simulink model "Project2"  (Simulink 8.0)
settings: Solver=ode23s  StartTime=0.0  StopTime=600  RelTol=1e-4
values from neighbouring files (symbols this model uses):
  a_1 = X(1)    [Init_Project1.m]
  a_2 = X(2)    [Init_Project1.m]
  a_3 = X(3)    [Init_Project1.m]
  A_max_wg = 0.035^2/4*pi    (= 0.000962112750162)    [Init_Project2.m]
  AFS = EngineMap.airfuel.AFs    [Init_Project1.m]
  alpha_REF_manual = 0    [Init_Project2.m]
  alphaEND = alphaINI    (= 0.1)    [Init_Project2.m]
  alphaINI = 0.1    [Init_Project2.m]
  alphaST = 0    [Init_Project2.m]
  BSR_max = turbin_efficiency_parameters(2)    [Init_Project2.m]
  c = sol(1)*(n_cyl/n_r)    [Init_Project1.m]
  C_d = x(3)    [Init_Project1.m]
  C_exh = mean(C_mat)    [Init_Project1.m]
  C_p = A\BMEP    [Init_Project2.m]
  c_p = cp_air    [Init_Project2.m]
  c_r1 = x(1)    [Init_Project1.m]
  c_r2 = x(2)    [Init_Project1.m]
  c_tc_fric = 1e-6    (= 1e-06)    [Init_Project2.m]
  Cd_wg = 0.9    [Init_Project2.m]
  comp_para2 = lsqcurvefit(fn2,[1 1 1 0.8 0.07 1.5], xdata, ydata)    [Init_Project2.m]
  cp_air = gamma_air*cv_air    (= 1213.33333333)    [Init_Project1.m]
  cp_exh = gamma_exh*cv_exh    (= 980)    [Init_Project1.m]
  cyl_sol = A\B    [Init_Project1.m]
  dC2 = 56e-03    (= 0.056)    [Init_Project2.m]
  dP_thrREF = 10e3    (= 10000)    [Init_Project2.m]
  dT1 = 52e-03    (= 0.052)    [Init_Project2.m]
  epsilon = 0.01    [Init_Project2.m]
  eta_T_max = turbin_efficiency_parameters(1)    [Init_Project2.m]
  gamma_air = 1.3    [Init_Project1.m]
  gamma_exh = 1.4    [Init_Project1.m]
  J_tc = 2.55e-5    (= 2.55e-05)    [Init_Project1.m]    (also in Init_Project2.m)
  k_inj = sol(1)    [Init_Project1.m]
  KiDriver = 0.02    [Init_Project1.m]
  KiFuel = 0.02    [Init_Project2.m]
  KpDriver = 0.04    [Init_Project1.m]
  KpFuel = 0.009    [Init_Project2.m]
  KpThr = 1e-6    (= 1e-06)    [Init_Project2.m]
  KpWg = 1e-6    (= 1e-06)    [Init_Project2.m]
  m_dot_c_corr_max = comp_para1(2)    [Init_Project2.m]
  n_cyl = 4    [Init_Project1.m]
  N_e_manual = 0    [Init_Project2.m]
  N_e_step = 1    [Init_Project2.m]
  n_r = 2    [Init_Project1.m]    (also in Init_Project2.m)
  n_vol_parameters = C\D    [Init_Project1.m]
  NEND = NINI    (= 2500)    [Init_Project2.m]
  NeRampInit = 800    [Init_Project2.m]
  NeSlope = 1    [Init_Project2.m]
  NeST = 30    [Init_Project2.m]
  NINI = 2500    [Init_Project2.m]
  p_amb = 101.3e3    (= 101300)    [Init_Project1.m]
  p_ref = comp.pCref    [Init_Project2.m]
  pedEND = 1    [Init_Project2.m]
  pedINI = 0    [Init_Project2.m]
  pedPos_manual = 0    [Init_Project2.m]
  pedST = 30    [Init_Project2.m]
  Psi_max = comp_para1(1)    [Init_Project2.m]
  q_HV = 44e6    (= 44000000)    [Init_Project1.m]
  R_air = 280    [Init_Project1.m]
  r_c = 9.3    [Init_Project1.m]
  R_exh = 280    [Init_Project1.m]
  rho_air = p_amb/(R_air*T_amb)    (= 1.23476352999)    [Init_Project1.m]
  t_0 = sol(2)/sol(1)    [Init_Project1.m]
  T_amb = 293    [Init_Project1.m]
  T_befthr = mean(T_befthr)    [Init_Project1.m]
  T_em = mean(T_em)    [Init_Project1.m]    (also in Init_Project2.m = turb.T03)
  T_ic = mean(T_amb./eta_c(1:34).*(Pi_c.^((gamma_air-1)/gamma_air)-ones(size(Pi_c))+eta_c(1:34)))    [Init_Project2.m]
  T_im = mean(T_im)    [Init_Project1.m]
  T_ref = comp.TCref    [Init_Project2.m]
  T_t = mean(T_em*(1-eta_T.*(1-Pi_T.^((gamma_exh-1)/gamma_exh))))    [Init_Project2.m]
  tau_d = 0.38    [Init_Project1.m]
  tau_mix = 0.1    [Init_Project1.m]
  Tau_th = T*3    [Init_Project1.m]
  tau_wg = 0.07    [Init_Project2.m]
  TFP_exp = turbine_parameters(2)    [Init_Project2.m]
  TFP_max = turbine_parameters(1)    [Init_Project2.m]
  TiThr = 0.1    [Init_Project2.m]
  TiWg = 1    [Init_Project2.m]
  V_D = 2.290 *10^-3    (= 0.00229)    [Init_Project1.m]    (also in Init_Project2.m = n_cyl*V_d)
  V_d = 2*a*pi*B^2/4    (= 0.000572555261117)    [Init_Project1.m]    (also in Init_Project2.m = B^2/4*pi*s)
  V_em = 2e-3    (= 0.002)    [Init_Project1.m]
  V_es = 10e-3    (= 0.01)    [Init_Project1.m]
  V_ic = 10e-3    (= 0.01)    [Init_Project2.m]
  V_im = 2e-3    (= 0.002)    [Init_Project1.m]
  VehicleArea = 2    [Init_Project1.m]
  VehicleMass = 1520    [Init_Project1.m]
  wg_REF_manual = 0    [Init_Project2.m]
  wgEND = wgINI    (= 1)    [Init_Project2.m]
  wgINI = 1    [Init_Project2.m]
  wgST = 30    [Init_Project2.m]
  WheelRadius = 0.3    [Init_Project1.m]
undefined symbols (not defined in the file or in its folder): magnitude, Newton, Raphson, TqEvsNe
libraries: simulink x1
(part 1 of 2)
settings Model: Creator=peran  LastModifiedBy=adalu838  ExtModeTrigMode=oneshot  ExtModeArmWhenConnect=off  ExtModeAutoUpdateStatusClock=off
settings DataIOCC: LimitDataPoints=off  SignalLoggingSaveFormat=ModelDataLogs  SignalLoggingName=sigsOut
settings OptimizationCC: BlockReduction=off  BooleanDataType=off  InitFltsAndDblsToZero=on
settings DebuggingCC: SaveWithParameterizedLinksMsg=none  SignalResolutionControl=TryResolveAllWithWarning  SolverPrmCheckMsg=none  MultiTaskDSMMsg=warning  MultiTaskCondExecSysMsg=none  FcnCallInpInsideContextMsg=UseLocalSettings  StrictBusMsg=None
settings HardwareCC: TargetUnknown=on
settings RTWCC: IncludeERTFirstTime=on
settings CodeAppCC: CustomSymbolStrType=$N$R$M_T  InternalIdentifier=Shortened
settings GRTTargetCC: TargetFcnLib=ansi_tfl_tmw.mat  ModelReferenceCompliant=off  CombineOutputUpdateFcns=off  MatFileLogging=off  GRTInterface=on

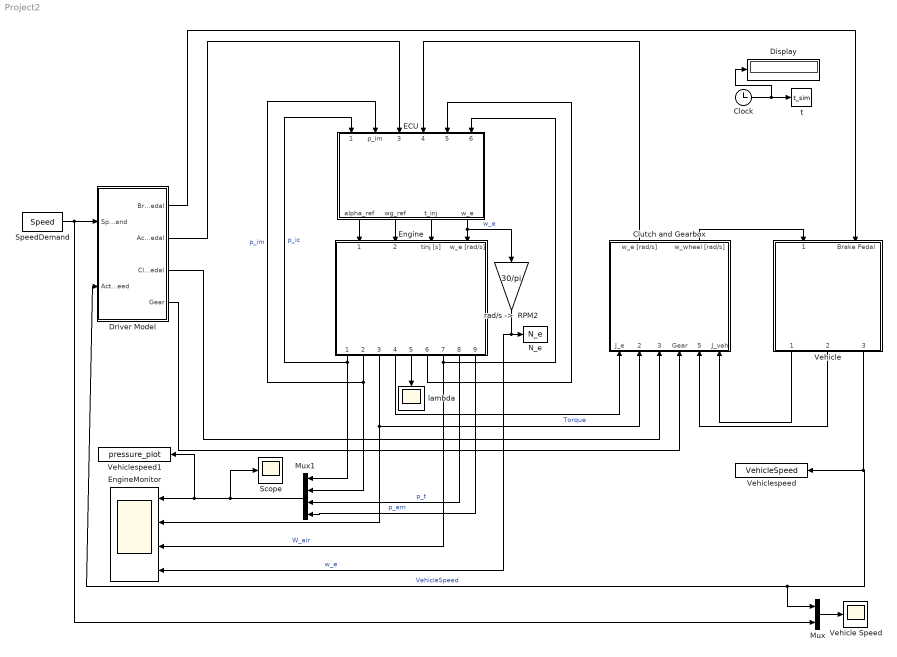
== system Project2 ==
  Clock : Clock
  Clutch and Gearbox : Subsystem
  Display : Display
  Driver Model : Subsystem
  ECU : Subsystem
  Engine : Subsystem
  EngineMonitor : Scope  NumInputPorts=4
      settings: ShowLegends=on  TimeRange=100  YMin=120000~137.25~0.09073~5780.2  YMax=330000~142.25~0.09094~5781.7  MaxDataPoints=3000
  Mux : Mux  Inputs=2
  Mux1 : Mux
  N_e : ToWorkspace  VariableName=N_e  SampleTime=-1
  Scope : Scope
      settings: ShowLegends=on  YMin=120000  YMax=330000  SaveName=ScopeData12
  SpeedDemand : FromWorkspace  VariableName=Speed  SampleTime=0
  Vehicle : Subsystem
  Vehicle Speed : Scope
      settings: ShowLegends=on  TimeRange=60  YMin=50  YMax=225  MaxDataPoints=3000
  Vehiclespeed : ToWorkspace  VariableName=VehicleSpeed  SampleTime=-1
  Vehiclespeed1 : ToWorkspace  VariableName=pressure_plot  SampleTime=-1
  lambda : Scope
      settings: TimeRange=600  YMin=-0.175  YMax=0  SaveName=ScopeData2  MaxDataPoints=3000
  "rad/s ->  RPM2" : Gain  Gain=30/pi  SaturateOnIntegerOverflow=on  OutDataTypeStr=Inherit: Same as input  ParamDataTypeStr=Inherit: Same as input
  t : ToWorkspace  VariableName=t_sim  SampleTime=-1
  wires:
  Vehicle/1(Vehicle Inertia [kgm^2]) -> Clutch and Gearbox/6(J_veh)
  Vehicle/2(Vehicle Torque [Nm]) -> Clutch and Gearbox/5(Tq_veh [Nm])
  Clutch and Gearbox/2(w_wheel [rad/s]) -> Vehicle/1(Wheel Speed [rad/s])
  Vehicle/3(Vehicle Speed[km/h]) -> Driver Model/2(Actual speed), Mux/1, Vehiclespeed/1  "VehicleSpeed"
  Driver Model/1(Brake Pedal) -> Vehicle/2(Brake Pedal)
  Driver Model/3(Clutch Pedal) -> Clutch and Gearbox/3(Clutch Pedal)
  Driver Model/2(Accelerator Pedal) -> ECU/3(ped_pos)
  Clutch and Gearbox/1(w_e [rad/s]) -> ECU/4(w_e [rad/s])
  SpeedDemand/1 -> Driver Model/1(Speed demand), Mux/2
  Driver Model/4(Gear) -> Clutch and Gearbox/4(Gear)
  Mux/1 -> Vehicle Speed/1
  Clock/1 -> t/1, Display/1
  Engine/7(m_dot_air [kg/s]) -> EngineMonitor/3, ECU/6(W_air [kg/s])  "W_air"
  Engine/6(Lambda Disc) -> ECU/5(lambdaDisc)
  Engine/2(p_im [Pa]) -> Mux1/2, ECU/2(p_im)  "p_im"
  Engine/4(J_e [kgm^2]) -> Clutch and Gearbox/1(J_e)
  Engine/3(Tq_e [Nm]) -> EngineMonitor/2, Clutch and Gearbox/2(Tq_e [Nm])  "Torque"
  Engine/1(p_ic [Pa]) -> Mux1/1, ECU/1(p_ic [Pa])  "p_ic"
  ECU/1(alpha_ref) -> Engine/1(alpha_REF [0..1])
  ECU/2(wg_ref) -> Engine/2(wg_REF [0..1])
  Mux1/1 -> Scope/1, Vehiclespeed1/1, EngineMonitor/1
  Engine/5(Lambda) -> lambda/1
  Engine/8(p_t [Pa]) -> Mux1/3  "p_t"
  Engine/9(p_em  [Pa]) -> Mux1/4  "p_em"
  ECU/4(w_e) -> Engine/4(w_e [rad/s]), "rad/s ->  RPM2"/1  "w_e"
  "rad/s ->  RPM2"/1 -> EngineMonitor/4, N_e/1  "w_e"
  ECU/3(t_inj) -> Engine/3(tinj [s])

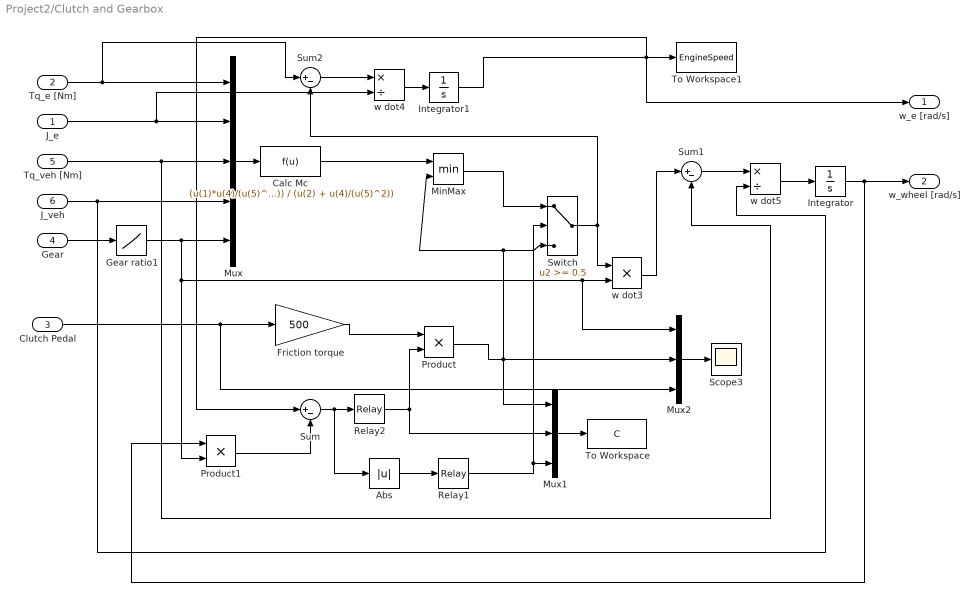
== system Project2/Clutch and Gearbox ==
  J_e : Inport
  Tq_e [Nm] : Inport  Port=2
  Clutch Pedal : Inport  Port=3
  Gear : Inport  Port=4
  Tq_veh [Nm] : Inport  Port=5
  J_veh : Inport  Port=6
  Abs : Abs  SaturateOnIntegerOverflow=on
  Calc Mc : Fcn  Expr=(u(1)*u(4)/(u(5)^2) + u(2)*u(3)/u(5)) / (u(2) + u(4)/(u(5)^2))
  Friction torque : Gain  Gain=500  SaturateOnIntegerOverflow=on  OutDataTypeStr=Inherit: Same as input  ParamDataTypeStr=Inherit: Same as input
  Gear ratio1 : Lookup  InputValues=[0:5]  Table=[30 16 7.5 4.5 3.2 2.5]  SaturateOnIntegerOverflow=on
  Integrator : Integrator
  Integrator1 : Integrator  InitialCondition=100  LimitOutput=on  LowerSaturationLimit=100
  MinMax : MinMax  Inputs=2  SaturateOnIntegerOverflow=on  InputSameDT=on
  Mux : Mux  Inputs=5
  Mux1 : Mux  Inputs=3
  Mux2 : Mux  Inputs=3
  Product : Product  SaturateOnIntegerOverflow=on  InputSameDT=on  OutDataTypeStr=Inherit: Same as first input
  Product1 : Product  SaturateOnIntegerOverflow=on  InputSameDT=on  OutDataTypeStr=Inherit: Same as first input
  Relay1 : Relay  OnSwitchValue=10  OffSwitchValue=1e-3  OnOutputValue=0  OffOutputValue=1
  Relay2 : Relay  OnSwitchValue=1e-1  OffSwitchValue=-1e-1  OffOutputValue=-1
  Scope3 : Scope
      settings: TimeRange=3.212851405622473  YMin=-1.88  YMax=-1.81
  Sum : Sum  Inputs=|+-  SaturateOnIntegerOverflow=on  InputSameDT=on  OutDataTypeStr=Inherit: Same as first input
  Sum1 : Sum  Inputs=|+-  SaturateOnIntegerOverflow=on  InputSameDT=on  OutDataTypeStr=Inherit: Same as first input
  Sum2 : Sum  Inputs=|+-  SaturateOnIntegerOverflow=on  InputSameDT=on  OutDataTypeStr=Inherit: Same as first input
  Switch : Switch  Threshold=0.5  SaturateOnIntegerOverflow=on  InputSameDT=on
  To Workspace : ToWorkspace  VariableName=C  SampleTime=-1  SaveFormat=Structure With Time
  To Workspace1 : ToWorkspace  VariableName=EngineSpeed  SampleTime=-1  SaveFormat=Structure With Time
  w dot3 : Product  Inputs=**  SaturateOnIntegerOverflow=on  InputSameDT=on  OutDataTypeStr=Inherit: Same as first input
  w dot4 : Product  Inputs=*/  SaturateOnIntegerOverflow=on  InputSameDT=on  OutDataTypeStr=Inherit: Same as first input
  w dot5 : Product  Inputs=*/  SaturateOnIntegerOverflow=on  InputSameDT=on  OutDataTypeStr=Inherit: Same as first input
  w_e [rad/s] : Outport
  w_wheel [rad/s] : Outport  Port=2
  wires:
  Switch/1 -> w dot3/1, Sum2/2
  Relay2/1 -> Mux1/2, Product/2
  Sum/1 -> Relay2/1, Abs/1
  Abs/1 -> Relay1/1
  MinMax/1 -> Switch/1
  Calc Mc/1 -> MinMax/1
  Mux/1 -> Calc Mc/1
  Mux2/1 -> Scope3/1
  Clutch Pedal/1 -> Friction torque/1, Mux2/3
  Tq_e [Nm]/1 -> Mux/1, Sum2/1
  J_e/1 -> Mux/2, w dot4/2
  Sum2/1 -> w dot4/1
  w dot4/1 -> Integrator1/1
  Integrator1/1 -> To Workspace1/1, w_e [rad/s]/1, Sum/1
  Relay1/1 -> Mux1/3, Switch/2
  Mux1/1 -> To Workspace/1
  Product1/1 -> Sum/2
  Product/1 -> Mux1/1, MinMax/2, Switch/3, Mux2/2
  Friction torque/1 -> Product/1
  Gear/1 -> Gear ratio1/1
  Gear ratio1/1 -> Product1/2, w dot3/2, Mux2/1, Mux/5
  w dot5/1 -> Integrator/1
  Sum1/1 -> w dot5/1
  Tq_veh [Nm]/1 -> Mux/3, Sum1/2
  J_veh/1 -> Mux/4, w dot5/2
  Integrator/1 -> w_wheel [rad/s]/1, Product1/1
  w dot3/1 -> Sum1/1

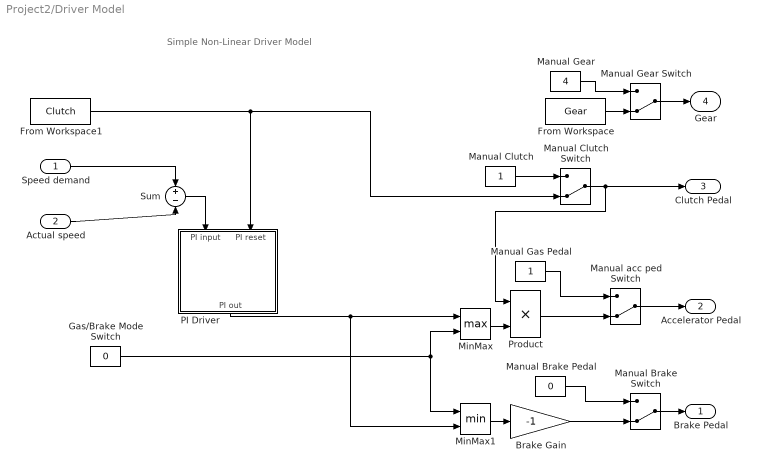
== system Project2/Driver Model ==
  note: Simple Non-Linear Driver Model
  Speed demand : Inport
  Actual speed : Inport  Port=2
  Brake Gain : Gain  Gain=-1  SaturateOnIntegerOverflow=on  OutDataTypeStr=Inherit: Same as input  ParamDataTypeStr=Inherit: Same as input
  From Workspace : FromWorkspace  VariableName=Gear  SampleTime=0
  From Workspace1 : FromWorkspace  VariableName=Clutch  SampleTime=0  OutputAfterFinalValue=Holding final value
  Gas/Brake Mode Switch : Constant  Value=0
  Manual Clutch : Constant
  Manual Gas Pedal : Constant
  Manual Gear : Constant  Value=4
  Manual Brake Pedal : Constant  Value=0
  Manual Brake Switch : ManualSwitch  CurrentSetting=0
  Manual Clutch Switch : ManualSwitch  CurrentSetting=0
  Manual Gear Switch : ManualSwitch  CurrentSetting=0
  Manual acc ped Switch : ManualSwitch  CurrentSetting=0
  MinMax : MinMax  Function=max  Inputs=2  SaturateOnIntegerOverflow=on  InputSameDT=on
  MinMax1 : MinMax  Inputs=2  SaturateOnIntegerOverflow=on  InputSameDT=on
  PI Driver : Subsystem
  Product : Product  SaturateOnIntegerOverflow=on  InputSameDT=on  OutDataTypeStr=Inherit: Same as first input
  Sum : Sum  Inputs=+-  SaturateOnIntegerOverflow=on  InputSameDT=on  OutDataTypeStr=Inherit: Same as first input
  Brake Pedal : Outport
  Accelerator Pedal : Outport  Port=2
  Clutch Pedal : Outport  Port=3
  Gear : Outport  Port=4
  wires:
  Product/1 -> Manual acc ped Switch/2
  MinMax/1 -> Product/2
  Manual acc ped Switch/1 -> Accelerator Pedal/1
  Manual Gas Pedal/1 -> Manual acc ped Switch/1
  Gas/Brake Mode Switch/1 -> MinMax1/1, MinMax/2
  MinMax1/1 -> Brake Gain/1
  PI Driver/1(PI out) -> MinMax1/2, MinMax/1
  From Workspace1/1 -> Manual Clutch Switch/2, PI Driver/2(PI reset)
  Manual Gear/1 -> Manual Gear Switch/1
  From Workspace/1 -> Manual Gear Switch/2
  Manual Gear Switch/1 -> Gear/1
  Manual Clutch/1 -> Manual Clutch Switch/1
  Brake Gain/1 -> Manual Brake Switch/2
  Manual Brake Pedal/1 -> Manual Brake Switch/1
  Manual Brake Switch/1 -> Brake Pedal/1
  Manual Clutch Switch/1 -> Clutch Pedal/1, Product/1
  Speed demand/1 -> Sum/1
  Sum/1 -> PI Driver/1(PI input)
  Actual speed/1 -> Sum/2

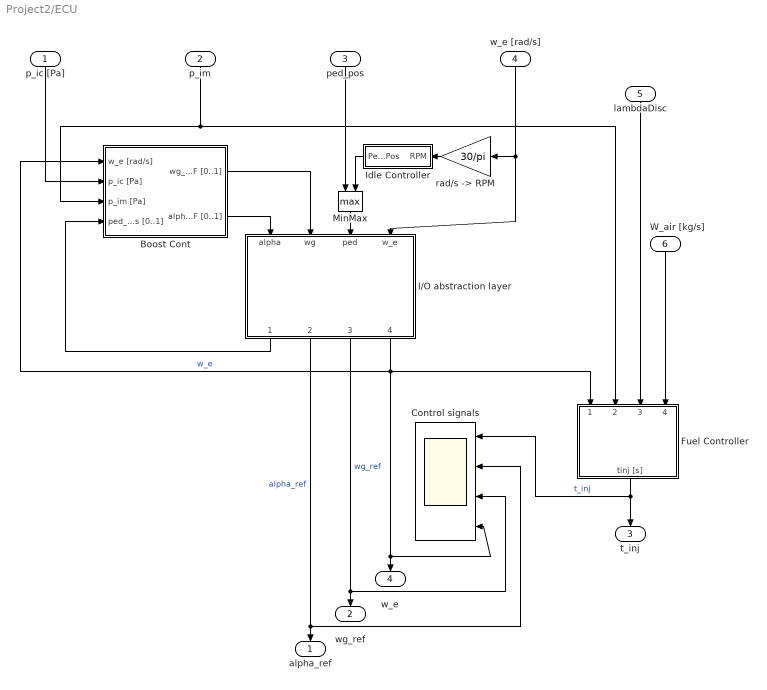
== system Project2/ECU ==
  p_ic [Pa] : Inport
  p_im : Inport  Port=2
  ped_pos : Inport  Port=3
  w_e [rad/s] : Inport  Port=4
  lambdaDisc : Inport  Port=5
  W_air [kg/s] : Inport  Port=6
  Boost Cont : Subsystem
  Control signals : Scope  NumInputPorts=4
      settings: TimeRange=65  YMin=0.0024~0.05~1~142  YMax=0.00335~0.0775~1~150.5  SaveName=ScopeData17  MaxDataPoints=3000
  Fuel Controller : Subsystem
  I/O abstraction layer : Subsystem
  Idle Controller : Subsystem
  MinMax : MinMax  Function=max  Inputs=2  SaturateOnIntegerOverflow=on  InputSameDT=on
  "rad/s -> RPM" : Gain  Gain=30/pi  SaturateOnIntegerOverflow=on  OutDataTypeStr=Inherit: Same as input  ParamDataTypeStr=Inherit: Same as input
  alpha_ref : Outport
  wg_ref : Outport  Port=2
  t_inj : Outport  Port=3
  w_e : Outport  Port=4
  wires:
  Idle Controller/1(PedalPos) -> MinMax/2
  Boost Cont/2(alpha_REF [0..1]) -> I/O abstraction layer/1(alpha)
  Boost Cont/1(wg_REF [0..1]) -> I/O abstraction layer/2(wg)
  MinMax/1 -> I/O abstraction layer/3(ped)
  I/O abstraction layer/1(pedPos [0..1]) -> Boost Cont/4(ped_pos [0..1])
  I/O abstraction layer/4(w_e [rad/s]) -> Fuel Controller/1(w_e [rad/s]), Boost Cont/1("w_e [rad/s] "), w_e/1, Control signals/4  "w_e"
  w_e [rad/s]/1 -> I/O abstraction layer/4(w_e), "rad/s -> RPM"/1
  W_air [kg/s]/1 -> Fuel Controller/4(W_air [kg/s])
  p_ic [Pa]/1 -> Boost Cont/2(p_ic [Pa])
  ped_pos/1 -> MinMax/1
  Fuel Controller/1(tinj [s]) -> t_inj/1, Control signals/1  "t_inj"
  I/O abstraction layer/2(alpha_REF [0..1]) -> alpha_ref/1, Control signals/2  "alpha_ref"
  I/O abstraction layer/3(wg_REF [0..100]) -> wg_ref/1, Control signals/3  "wg_ref"
  lambdaDisc/1 -> Fuel Controller/3(lambdaDisc)
  p_im/1 -> Fuel Controller/2(p_im [Pa]), Boost Cont/3(p_im [Pa])
  "rad/s -> RPM"/1 -> Idle Controller/1(RPM)

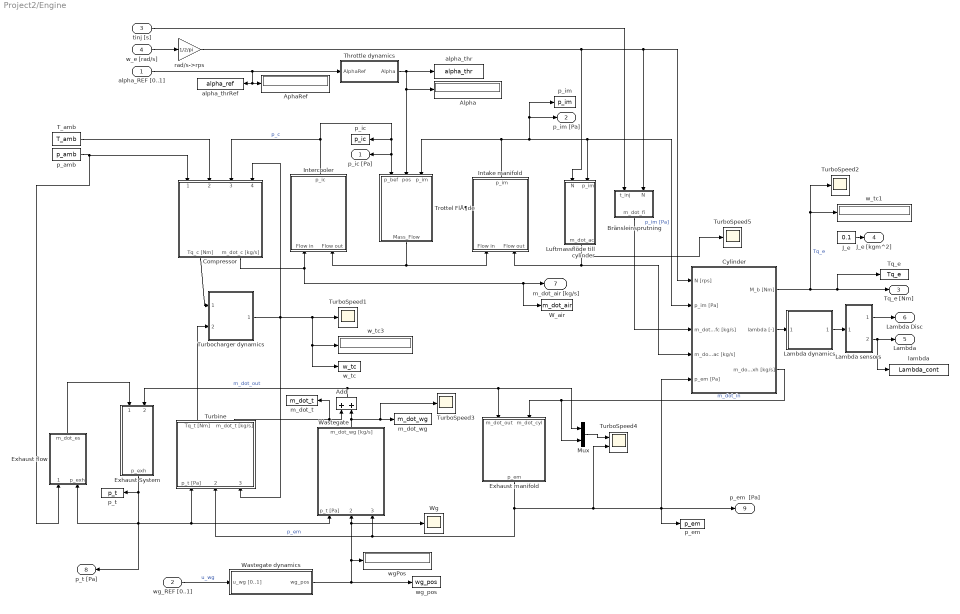
== system Project2/Engine ==
  alpha_REF [0..1] : Inport
  wg_REF [0..1] : Inport  Port=2
  tinj [s] : Inport  Port=3
  w_e [rad/s] : Inport  Port=4
  Add : Sum
  Alpha : Display
  AphaRef : Display
  Bränsleinsprutning : Subsystem
  Compressor : Subsystem
  Cylinder : Subsystem
  Exhaust System : Subsystem
  Exhaust flow : Subsystem
  Exhaust manifold : Subsystem
  Intake manifold : Subsystem
  Intercooler : Subsystem
  J_e : Constant  Value=0.1
  Lambda dynamics : Subsystem
  Lambda sensors : Subsystem
  Luftmassflöde till cylinder : Subsystem
  Mux : Mux  Inputs=2
  T_amb : Constant  Value=T_amb
  Throttle dynamics : Subsystem
  Tq_e : ToWorkspace  VariableName=Tq_e  SampleTime=-1
  Trottel FlÃ¶de : Subsystem
  Turbine : Subsystem
  TurboSpeed{1..3,5} (4 alike) : Scope
      TurboSpeed1 settings: TimeRange=100  YMin=2000  YMax=21000  SaveName=ScopeData3
      TurboSpeed2 settings: TimeRange=100  YMin=2000  YMax=21000  SaveName=ScopeData22
      TurboSpeed3 settings: TimeRange=100  YMin=2000  YMax=21000  SaveName=ScopeData23
      TurboSpeed5 settings: TimeRange=60  YMin=0.002  YMax=0.011  SaveName=ScopeData25
  TurboSpeed4 : Scope  NumInputPorts=2
      settings: ShowLegends=on  TimeRange=60  YMin=0.002~0.002  YMax=0.012~0.012  SaveName=ScopeData24
  Turbocharger dynamics : Subsystem
  W_air : ToWorkspace  VariableName=m_dot_air  SampleTime=-1
  Wastegate : Subsystem
  Wastegate dynamics : Subsystem
  Wg : Scope
      settings: TimeRange=100  YMin=0.7  YMax=1.025  SaveName=ScopeData9
  alpha_thr : ToWorkspace  VariableName=alpha_thr  SampleTime=-1
  alpha_thrRef : ToWorkspace  VariableName=alpha_ref  SampleTime=-1
  lambda : ToWorkspace  VariableName=Lambda_cont  SampleTime=-1
  m_dot_t : ToWorkspace  VariableName=m_dot_t  SampleTime=-1
  m_dot_wg : ToWorkspace  VariableName=m_dot_wg  SampleTime=-1
  p_amb : Constant  Value=p_amb
  p_em : ToWorkspace  VariableName=p_em  SampleTime=-1
  p_ic : ToWorkspace  VariableName=p_ic  SampleTime=-1
  p_im : ToWorkspace  VariableName=p_im  SampleTime=-1
  p_t : ToWorkspace  VariableName=p_t  SampleTime=-1
  rad/s->rps : Gain  Gain=1/2/pi
  w_tc : ToWorkspace  VariableName=w_tc  SampleTime=-1
  w_tc1 : Display
  w_tc3 : Display
  wgPos : Display
  wg_pos : ToWorkspace  VariableName=wg_pos  SampleTime=-1
  p_ic [Pa] : Outport
  p_im [Pa] : Outport  Port=2
  Tq_e [Nm] : Outport  Port=3
  J_e [kgm^2] : Outport  Port=4
  Lambda : Outport  Port=5
  Lambda Disc : Outport  Port=6
  m_dot_air [kg/s] : Outport  Port=7
  p_t [Pa] : Outport  Port=8
  p_em  [Pa] : Outport  Port=9
  wires:
  J_e/1 -> J_e [kgm^2]/1
  Lambda sensors/1(lam_d) -> Lambda Disc/1
  Lambda sensors/2(lam_c) -> Lambda/1, lambda/1
  Lambda dynamics/1(lam_bc) -> Lambda sensors/1(lam)
  T_amb/1 -> Compressor/2(T_amb [K])
  p_amb/1 -> Compressor/1(p_amb [Pa]), Exhaust flow/1(p_amb)
  Compressor/2(m_dot_c [kg/s]) -> Intercooler/1(Flow in), m_dot_air [kg/s]/1, W_air/1
  Trottel FlÃ¶de/1(Mass_Flow) -> Intercooler/2(Flow out), Intake manifold/1(Flow in)
  Intercooler/1(p_ic) -> Compressor/3("p_ic [Pa] "), p_ic/1, p_ic [Pa]/1, Trottel FlÃ¶de/1(p_bef)  "p_c"
  Intake manifold/1(p_im) -> Trottel FlÃ¶de/3(p_im), Luftmassflöde till cylinder/2(p_im), Cylinder/2(p_im [Pa]), p_im [Pa]/1, p_im/1  "p_im [Pa]"
  Throttle dynamics/1(Alpha) -> Trottel FlÃ¶de/2(pos), Alpha/1, alpha_thr/1
  alpha_REF [0..1]/1 -> Throttle dynamics/1(AlphaRef), AphaRef/1, alpha_thrRef/1
  Turbocharger dynamics/1(w_tc [rad/s]) -> Turbine/3(w_tc [rad/s]), w_tc/1, w_tc3/1, TurboSpeed1/1, Compressor/4(w_tc [rad/s])
  Compressor/1(Tq_c [Nm]) -> Turbocharger dynamics/1(Tq_c [Nm])
  Luftmassflöde till cylinder/1(m_dot_ac) -> TurboSpeed5/1, Cylinder/4(m_dot_ac [kg/s]), Intake manifold/2("Flow out ")
  rad/s->rps/1 -> Cylinder/1(N [rps]), Bränsleinsprutning/2(N), Luftmassflöde till cylinder/1(N)
  Bränsleinsprutning/1(m_dot_fi) -> Cylinder/3(m_dot_fc [kg/s])
  Cylinder/3(m_dot_exh [kg/s]) -> Mux/2, Exhaust manifold/2(m_dot_cyl)  "m_dot_in"
  Cylinder/1(M_b [Nm]) -> TurboSpeed2/1, w_tc1/1, Tq_e [Nm]/1, Tq_e/1  "Tq_e"
  Cylinder/2(lambda [-]) -> Lambda dynamics/1(lam_cyl)
  Turbine/2(m_dot_t [kg/s]) -> Add/1, m_dot_t/1
  Wastegate/1(m_dot_wg [kg/s]) -> TurboSpeed3/1, m_dot_wg/1, Add/2
  Add/1 -> Exhaust manifold/1("m_dot_out "), Mux/1, Exhaust System/2(Flow in)  "m_dot_out"
  Exhaust System/1(p_exh) -> p_t/1, p_t [Pa]/1, Wastegate/1(p_t [Pa]), Turbine/1("p_t [Pa] "), Exhaust flow/2(p_exh)
  Wastegate dynamics/1(wg_pos) -> wg_pos/1, wgPos/1, Wg/1, Wastegate/2(wg_pos [0..1])
  wg_REF [0..1]/1 -> Wastegate dynamics/1(u_wg [0..1])  "u_wg"
  Exhaust flow/1(m_dot_es) -> Exhaust System/1("Flow out ")
  Exhaust manifold/1(p_em) -> p_em/1, Cylinder/5(p_em [Pa]), p_em  [Pa]/1, TurboSpeed4/2, Turbine/2(p_em [Pa]), Wastegate/3(p_em [Pa])  "p_em"
  tinj [s]/1 -> Bränsleinsprutning/1(t_inj)
  Turbine/1(Tq_t [Nm]) -> Turbocharger dynamics/2(Tq_t [Nm])
  w_e [rad/s]/1 -> rad/s->rps/1
  Mux/1 -> TurboSpeed4/1

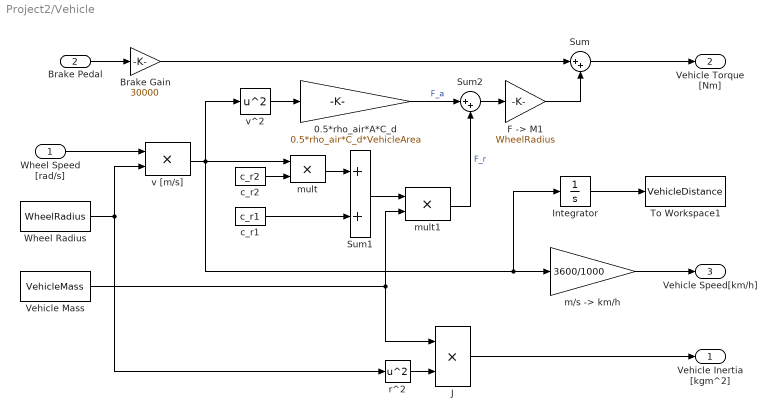
== system Project2/Vehicle ==
  Wheel Speed [rad/s] : Inport
  Brake Pedal : Inport  Port=2
  0.5*rho_air*A*C_d : Gain  Gain=0.5*rho_air*C_d*VehicleArea  SaturateOnIntegerOverflow=on  OutDataTypeStr=Inherit: Same as input  ParamDataTypeStr=Inherit: Same as input
  Brake Gain : Gain  Gain=30000  SaturateOnIntegerOverflow=on  OutDataTypeStr=Inherit: Same as input  ParamDataTypeStr=Inherit: Same as input
  "F -> M1" : Gain  Gain=WheelRadius  SaturateOnIntegerOverflow=on  OutDataTypeStr=Inherit: Same as input  ParamDataTypeStr=Inherit: Same as input
  Integrator : Integrator
  J : Product  SaturateOnIntegerOverflow=on  OutDataTypeStr=Inherit: Same as first input
  Sum : Sum  Inputs=|++  SaturateOnIntegerOverflow=on
  Sum1 : Sum  SaturateOnIntegerOverflow=on
  Sum2 : Sum  Inputs=|++  SaturateOnIntegerOverflow=on
  To Workspace1 : ToWorkspace  VariableName=VehicleDistance  SampleTime=-1
  Vehicle Mass : Constant  Value=VehicleMass
  Wheel Radius : Constant  Value=WheelRadius
  c_r1 : Constant  Value=c_r1
  c_r2 : Constant  Value=c_r2
  "m/s -> km/h" : Gain  Gain=3600/1000  SaturateOnIntegerOverflow=on  OutDataTypeStr=Inherit: Same as input  ParamDataTypeStr=Inherit: Same as input
  mult : Product  SaturateOnIntegerOverflow=on  OutDataTypeStr=Inherit: Same as first input
  mult1 : Product  SaturateOnIntegerOverflow=on  OutDataTypeStr=Inherit: Same as first input
  r^2 : Math  Operator=square  SaturateOnIntegerOverflow=on
  v [m/s] : Product  SaturateOnIntegerOverflow=on  OutDataTypeStr=Inherit: Same as first input
  v^2 : Math  Operator=square  SaturateOnIntegerOverflow=on
  Vehicle Inertia [kgm^2] : Outport
  Vehicle Torque [Nm] : Outport  Port=2
  Vehicle Speed[km/h] : Outport  Port=3
  wires:
  Brake Pedal/1 -> Brake Gain/1
  Wheel Radius/1 -> v [m/s]/2, r^2/1
  v [m/s]/1 -> Integrator/1, "m/s -> km/h"/1, mult/1, v^2/1
  "m/s -> km/h"/1 -> Vehicle Speed[km/h]/1
  Brake Gain/1 -> Sum/1
  Sum/1 -> Vehicle Torque [Nm]/1
  r^2/1 -> J/2
  Vehicle Mass/1 -> mult1/2, J/1
  J/1 -> Vehicle Inertia [kgm^2]/1
  Integrator/1 -> To Workspace1/1
  Wheel Speed [rad/s]/1 -> v [m/s]/1
  c_r2/1 -> mult/2
  mult/1 -> Sum1/1
  c_r1/1 -> Sum1/2
  Sum1/1 -> mult1/1
  mult1/1 -> Sum2/2  "F_r"
  v^2/1 -> 0.5*rho_air*A*C_d/1
  0.5*rho_air*A*C_d/1 -> Sum2/1  "F_a"
  Sum2/1 -> "F -> M1"/1
  "F -> M1"/1 -> Sum/2

== system Project2/Driver Model/PI Driver ==
  PI input : Inport
  PI reset : Inport  Port=2
  Integrator : Integrator  ExternalReset=either  LimitOutput=on  UpperSaturationLimit=30  LowerSaturationLimit=0
  Ki : Gain  Gain=KiDriver  SaturateOnIntegerOverflow=on  OutDataTypeStr=Inherit: Same as input  ParamDataTypeStr=Inherit: Same as input
  Kp : Gain  Gain=KpDriver  SaturateOnIntegerOverflow=on  OutDataTypeStr=Inherit: Same as input  ParamDataTypeStr=Inherit: Same as input
  Saturation : Saturate  UpperLimit=1  LowerLimit=-1
  Sum : Sum  Inputs=|++  SaturateOnIntegerOverflow=on  InputSameDT=on  OutDataTypeStr=Inherit: Same as first input
  PI out : Outport
  wires:
  PI input/1 -> Kp/1, Integrator/1
  Integrator/1 -> Ki/1
  Ki/1 -> Sum/2
  Sum/1 -> Saturation/1
  Saturation/1 -> PI out/1
  PI reset/1 -> Integrator/2
  Kp/1 -> Sum/1

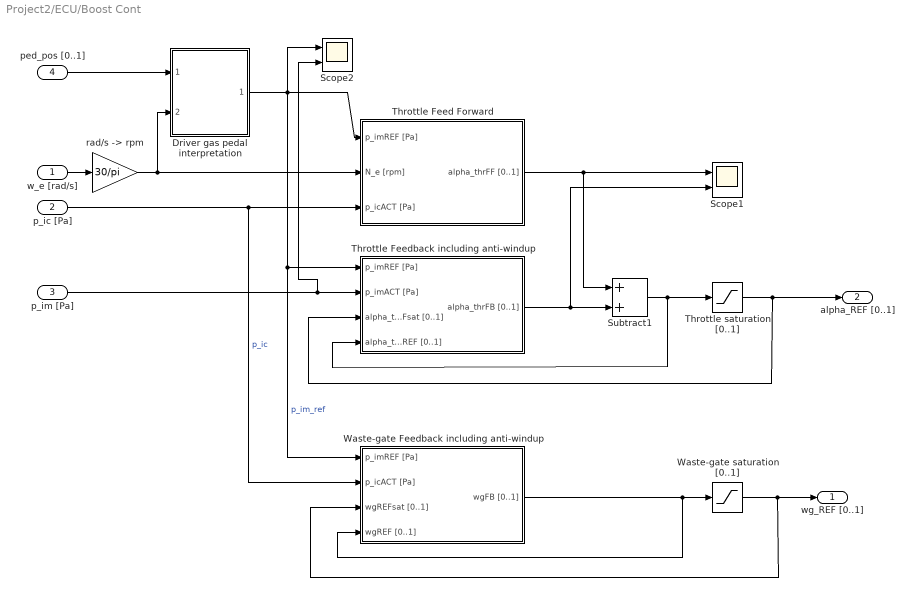
== system Project2/ECU/Boost Cont ==
  "w_e [rad/s] " : Inport
  p_ic [Pa] : Inport  Port=2
  p_im [Pa] : Inport  Port=3
  ped_pos [0..1] : Inport  Port=4
  Driver gas pedal interpretation : Subsystem
  Scope1 : Scope  NumInputPorts=2
      settings: ShowLegends=on  YMin=-1.73472e-17~-0.07  YMax=0.24~6.93889e-18  SaveName=ScopeData18
  Scope2 : Scope  NumInputPorts=2
      settings: ShowLegends=on  YMin=10000~15000  YMax=95000~105000  SaveName=ScopeData20
  Subtract1 : Sum
  Throttle saturation [0..1] : Saturate  UpperLimit=1  LowerLimit=0
  Throttle Feed Forward : Subsystem
  Throttle Feedback including anti-windup : Subsystem
  Waste-gate saturation [0..1] : Saturate  UpperLimit=1  LowerLimit=0
  Waste-gate Feedback including anti-windup : Subsystem
  "rad/s -> rpm" : Gain  Gain=30/pi  SaturateOnIntegerOverflow=on  OutDataTypeStr=Inherit: Same as input  ParamDataTypeStr=Inherit: Same as input
  wg_REF [0..1] : Outport
  alpha_REF [0..1] : Outport  Port=2
  wires:
  ped_pos [0..1]/1 -> Driver gas pedal interpretation/1(ped_pos [0..1])
  Driver gas pedal interpretation/1(p_im_ref) -> Scope2/1, Throttle Feed Forward/1(p_imREF [Pa]), Throttle Feedback including anti-windup/1(p_imREF [Pa]), Waste-gate Feedback including anti-windup/1(p_imREF [Pa])  "p_im_ref"
  Throttle Feed Forward/1(alpha_thrFF [0..1]) -> Scope1/1, Subtract1/1
  Throttle Feedback including anti-windup/1(alpha_thrFB [0..1]) -> Scope1/2, Subtract1/2
  Subtract1/1 -> Throttle saturation [0..1]/1, Throttle Feedback including anti-windup/4(alpha_thrREF [0..1])
  p_im [Pa]/1 -> Scope2/2, Throttle Feedback including anti-windup/2(p_imACT [Pa])
  "w_e [rad/s] "/1 -> "rad/s -> rpm"/1
  "rad/s -> rpm"/1 -> Throttle Feed Forward/2(N_e [rpm]), Driver gas pedal interpretation/2(N_e [rpm])
  p_ic [Pa]/1 -> Throttle Feed Forward/3(p_icACT [Pa]), Waste-gate Feedback including anti-windup/2(p_icACT [Pa])  "p_ic"
  Throttle saturation [0..1]/1 -> Throttle Feedback including anti-windup/3(alpha_thrREFsat [0..1]), alpha_REF [0..1]/1
  Waste-gate saturation [0..1]/1 -> wg_REF [0..1]/1, Waste-gate Feedback including anti-windup/3(wgREFsat [0..1])
  Waste-gate Feedback including anti-windup/1(wgFB [0..1]) -> Waste-gate saturation [0..1]/1, Waste-gate Feedback including anti-windup/4(wgREF [0..1])

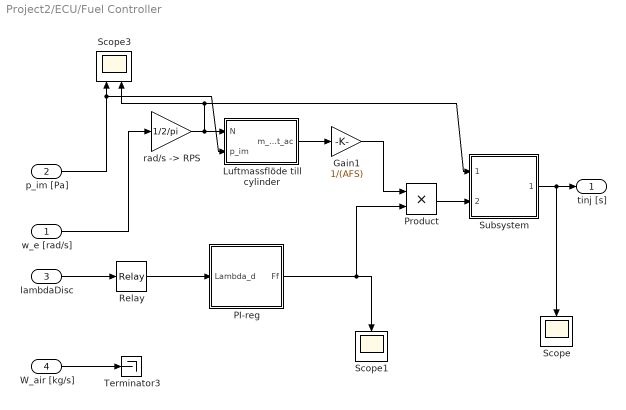
== system Project2/ECU/Fuel Controller ==
  w_e [rad/s] : Inport
  p_im [Pa] : Inport  Port=2
  lambdaDisc : Inport  Port=3
  W_air [kg/s] : Inport  Port=4
  Gain1 : Gain  Gain=1/(AFS)
  Luftmassflöde till cylinder : Subsystem
  PI-reg : Subsystem
  Product : Product  RndMeth=Zero
  Relay : Relay  OnSwitchValue=1  OffSwitchValue=0  OffOutputValue=-1
  Scope : Scope
      settings: SaveName=ScopeData10
  Scope1 : Scope
      settings: SaveName=ScopeData6
  Scope3 : Scope  NumInputPorts=2
      settings: YMin=-5~-5  YMax=5~5  SaveName=ScopeData16
  Subsystem : Subsystem
  Terminator3 : Terminator
  "rad/s -> RPS" : Gain  Gain=1/2/pi  SaturateOnIntegerOverflow=on  OutDataTypeStr=Inherit: Same as input  ParamDataTypeStr=Inherit: Same as input
  tinj [s] : Outport
  wires:
  W_air [kg/s]/1 -> Terminator3/1
  w_e [rad/s]/1 -> "rad/s -> RPS"/1
  p_im [Pa]/1 -> Luftmassflöde till cylinder/2(p_im), Scope3/1
  lambdaDisc/1 -> Relay/1
  "rad/s -> RPS"/1 -> Luftmassflöde till cylinder/1(N), Subsystem/1(Varvtal), Scope3/2
  Subsystem/1(t_injref) -> Scope/1, tinj [s]/1
  Luftmassflöde till cylinder/1(m_dot_ac) -> Gain1/1
  Product/1 -> Subsystem/2(m_dotref)
  Gain1/1 -> Product/1
  Relay/1 -> PI-reg/1(Lambda_d)
  PI-reg/1(Ff) -> Scope1/1, Product/2

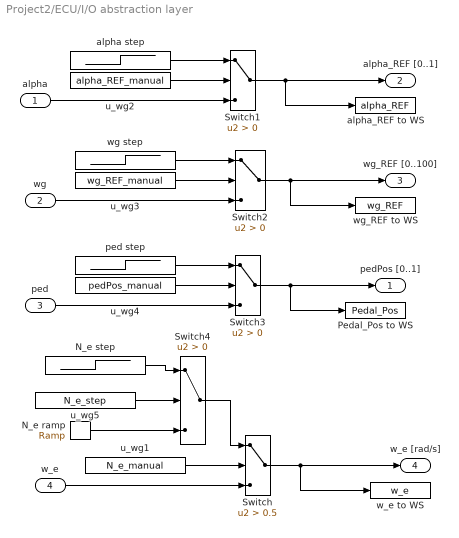
== system Project2/ECU/I/O abstraction layer ==
  alpha : Inport
  wg : Inport  Port=2
  ped : Inport  Port=3
  w_e : Inport  Port=4
  N_e ramp : simulink/Sources/Ramp  slope=NeSlope*pi/30  start=NeStartTime  X0=NeRampInit*pi/30
  N_e step : Step  Time=NeST  Before=NINI*pi/30  After=NEND*pi/30  SampleTime=0
  Pedal_Pos to WS : ToWorkspace  VariableName=Pedal_Pos  SampleTime=-1
  Switch : Switch  Criteria=u2 > Threshold  Threshold=0.5
  Switch{1..4} (4 alike) : Switch  Criteria=u2 > Threshold
  alpha step : Step  Time=alphaST  Before=alphaINI  After=alphaEND  SampleTime=0
  alpha_REF to WS : ToWorkspace  VariableName=alpha_REF  SampleTime=-1
  ped step : Step  Time=pedST  Before=pedINI  After=pedEND  SampleTime=0
  u_wg1 : Constant  Value=N_e_manual
  u_wg2 : Constant  Value=alpha_REF_manual
  u_wg3 : Constant  Value=wg_REF_manual
  u_wg4 : Constant  Value=pedPos_manual
  u_wg5 : Constant  Value=N_e_step
  w_e to WS : ToWorkspace  VariableName=w_e  SampleTime=-1
  wg step : Step  Time=wgST  Before=wgINI  After=wgEND  SampleTime=0
  wg_REF to WS : ToWorkspace  VariableName=wg_REF  SampleTime=-1
  pedPos [0..1] : Outport
  alpha_REF [0..1] : Outport  Port=2
  wg_REF [0..100] : Outport  Port=3
  w_e [rad/s] : Outport  Port=4
  wires:
  Switch/1 -> w_e [rad/s]/1, w_e to WS/1
  u_wg1/1 -> Switch/2
  w_e/1 -> Switch/3
  Switch1/1 -> alpha_REF [0..1]/1, alpha_REF to WS/1
  alpha step/1 -> Switch1/1
  u_wg2/1 -> Switch1/2
  alpha/1 -> Switch1/3
  Switch2/1 -> wg_REF [0..100]/1, wg_REF to WS/1
  wg step/1 -> Switch2/1
  u_wg3/1 -> Switch2/2
  wg/1 -> Switch2/3
  Switch3/1 -> pedPos [0..1]/1, Pedal_Pos to WS/1
  ped step/1 -> Switch3/1
  u_wg4/1 -> Switch3/2
  ped/1 -> Switch3/3
  N_e step/1 -> Switch4/1
  Switch4/1 -> Switch/1
  N_e ramp/1 -> Switch4/3
  u_wg5/1 -> Switch4/2

== system Project2/ECU/Idle Controller ==
  RPM : Inport
  Constant : Constant  Value=800
  Gain : Gain  Gain=1/40000  SaturateOnIntegerOverflow=on  OutDataTypeStr=Inherit: Same as input  ParamDataTypeStr=Inherit: Same as input
  Saturation : Saturate  UpperLimit=1  LowerLimit=0
  Sum : Sum  Inputs=-+  SaturateOnIntegerOverflow=on  InputSameDT=on  OutDataTypeStr=Inherit: Same as first input
  PedalPos : Outport
  wires:
  RPM/1 -> Sum/1
  Constant/1 -> Sum/2
  Saturation/1 -> PedalPos/1
  Gain/1 -> Saturation/1
  Sum/1 -> Gain/1

== system Project2/Engine/Bränsleinsprutning ==
  t_inj : Inport
  N : Inport  Port=2
  Add : Sum  Inputs=+-
  Constant : Constant  Value=0
  MinMax : MinMax  Function=max  Inputs=2
  Product : Product  RndMeth=Zero
  c1 : Gain  Gain=k_inj*(n_cyl/n_r)
  t_0 : Constant  Value=t_0
  m_dot_fi : Outport
  wires:
  t_0/1 -> Add/2
  Add/1 -> Product/1
  N/1 -> Product/2
  c1/1 -> m_dot_fi/1
  MinMax/1 -> c1/1
  Product/1 -> MinMax/1
  Constant/1 -> MinMax/2
  t_inj/1 -> Add/1

== system Project2/Engine/Compressor ==
  p_amb [Pa] : Inport
  T_amb [K] : Inport  Port=2
  "p_ic [Pa] " : Inport  Port=3
  w_tc [rad/s] : Inport  Port=4
  Pi_c : Product  Inputs=*/
  Subsystem : Subsystem
  Subsystem2 : Subsystem
  Subsystem3 : Subsystem
  Subsystem4 : Subsystem
  Subsystem5 : Subsystem
  To Workspace : ToWorkspace  VariableName=PiC_model  SampleTime=-1
  To Workspace1 : ToWorkspace  VariableName=WcCorr_model  SampleTime=-1
  Tq_c [Nm] : Outport
  m_dot_c [kg/s] : Outport  Port=2
  wires:
  "p_ic [Pa] "/1 -> Pi_c/1
  p_amb [Pa]/1 -> Subsystem2/3(p_amb), Pi_c/2
  Pi_c/1 -> To Workspace/1, Subsystem/2(Pi_c), Subsystem3/3(Pi_c), Subsystem5/1(Pi_c)
  T_amb [K]/1 -> Subsystem/3(T_amb), Subsystem3/2(T01), Subsystem4/1(T01), Subsystem2/2(T_amb)
  w_tc [rad/s]/1 -> Subsystem/1(Nc_corr), Subsystem4/4(w_tc)
  Subsystem/1(m_dot_c_corr) -> To Workspace1/1, Subsystem5/2(m_dot_ccorr), Subsystem2/1(m_dot_corr)
  Subsystem2/1(m_dot_c) -> Subsystem4/3(mdot_c), m_dot_c [kg/s]/1
  Subsystem4/1(Tq_c) -> Tq_c [Nm]/1
  Subsystem5/1(eta_c) -> Subsystem3/1(eta_c)
  Subsystem3/1(T_c) -> Subsystem4/2(T02)

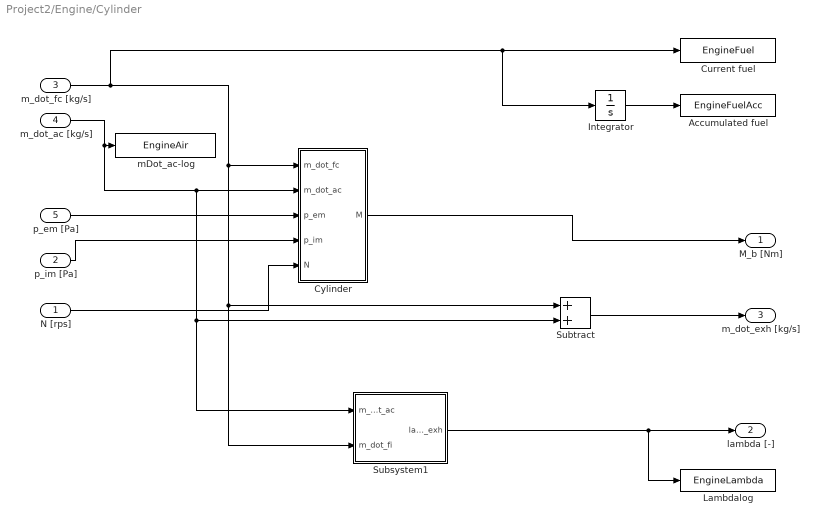
== system Project2/Engine/Cylinder ==
  N [rps] : Inport
  p_im [Pa] : Inport  Port=2
  m_dot_fc [kg/s] : Inport  Port=3
  m_dot_ac [kg/s] : Inport  Port=4
  p_em [Pa] : Inport  Port=5
  Accumulated fuel : ToWorkspace  VariableName=EngineFuelAcc  SampleTime=-1
  Current fuel : ToWorkspace  VariableName=EngineFuel  SampleTime=-1
  Cylinder : Subsystem
  Integrator : Integrator
  Lambdalog : ToWorkspace  VariableName=EngineLambda  SampleTime=-1
  Subsystem1 : Subsystem
  Subtract : Sum
  mDot_ac-log : ToWorkspace  VariableName=EngineAir  SampleTime=-1
  M_b [Nm] : Outport
  lambda [-] : Outport  Port=2
  m_dot_exh [kg/s] : Outport  Port=3
  wires:
  Integrator/1 -> Accumulated fuel/1
  m_dot_fc [kg/s]/1 -> Subtract/1, Subsystem1/2(m_dot_fi), Cylinder/1(m_dot_fc), Current fuel/1, Integrator/1
  m_dot_ac [kg/s]/1 -> Subsystem1/1(m_dot_ac), Subtract/2, Cylinder/2(m_dot_ac), mDot_ac-log/1
  Subsystem1/1(lambda_exh) -> Lambdalog/1, lambda [-]/1
  Subtract/1 -> m_dot_exh [kg/s]/1
  p_em [Pa]/1 -> Cylinder/3(p_em)
  p_im [Pa]/1 -> Cylinder/4(p_im)
  N [rps]/1 -> Cylinder/5(N)
  Cylinder/1(M) -> M_b [Nm]/1

== system Project2/Engine/Exhaust System ==
  "Flow out " : Inport
  Flow in : Inport  Port=2
  Integrator : Integrator  InitialCondition=103e3
  Product : Product  Inputs=***/  SaturateOnIntegerOverflow=on  OutDataTypeStr=Inherit: Same as first input
  R : Constant  Value=R_exh
  Scope : Scope  NumInputPorts=2
      settings: YMin=-5~-5  YMax=5~5  SaveName=ScopeData8
  Sum : Sum  Inputs=|+-  SaturateOnIntegerOverflow=on
  T_t : Constant  Value=T_t
  V_es : Constant  Value=V_es
  p_exh : Outport
  wires:
  V_es/1 -> Product/4
  Sum/1 -> Product/1
  T_t/1 -> Product/3
  R/1 -> Product/2
  "Flow out "/1 -> Scope/2, Sum/2
  Flow in/1 -> Scope/1, Sum/1
  Product/1 -> Integrator/1
  Integrator/1 -> p_exh/1

== system Project2/Engine/Exhaust flow ==
  p_amb : Inport
  p_exh : Inport  Port=2
  Constant1 : Constant  Value=0
  Gain : Gain  Gain=1/(T_em*R_exh*C_exh)
  MinMax : MinMax  Function=max  Inputs=2
  Product : Product  RndMeth=Zero
  Scope : Scope  NumInputPorts=2
      settings: YMin=-5~-5  YMax=5~5  SaveName=ScopeData4
  Sqrt : Sqrt  SaturateOnIntegerOverflow=on
  Subtract : Sum  Inputs=+-
  m_dot_es : Outport
  wires:
  Sqrt/1 -> m_dot_es/1
  p_exh/1 -> Product/1, Scope/1, Subtract/1
  p_amb/1 -> Scope/2, Subtract/2
  Subtract/1 -> Gain/1
  Gain/1 -> Product/2
  Constant1/1 -> MinMax/1
  Product/1 -> MinMax/2
  MinMax/1 -> Sqrt/1

== system Project2/Engine/Exhaust manifold ==
  "m_dot_out " : Inport
  m_dot_cyl : Inport  Port=2
  Integrator : Integrator  InitialCondition=106e3
  Product : Product  Inputs=***/  SaturateOnIntegerOverflow=on  OutDataTypeStr=Inherit: Same as first input
  R : Constant  Value=R_exh
  Sum : Sum  Inputs=|+-  SaturateOnIntegerOverflow=on
  T_im : Constant  Value=T_em
  V_im : Constant  Value=V_em
  p_em : Outport
  wires:
  Product/1 -> Integrator/1
  V_im/1 -> Product/4
  Sum/1 -> Product/1
  T_im/1 -> Product/3
  R/1 -> Product/2
  "m_dot_out "/1 -> Sum/2
  m_dot_cyl/1 -> Sum/1
  Integrator/1 -> p_em/1

== system Project2/Engine/Intake manifold ==
  Flow in : Inport
  "Flow out " : Inport  Port=2
  Integrator : Integrator  InitialCondition=p_amb/2  LowerSaturationLimit=0
  Product : Product  Inputs=***/  SaturateOnIntegerOverflow=on  OutDataTypeStr=Inherit: Same as first input
  R : Constant  Value=R_air
  Sum : Sum  Inputs=|+-  SaturateOnIntegerOverflow=on
  T_im : Constant  Value=T_im
  V_im : Constant  Value=V_im
  p_im : Outport
  wires:
  Product/1 -> Integrator/1
  V_im/1 -> Product/4
  Sum/1 -> Product/1
  T_im/1 -> Product/3
  R/1 -> Product/2
  "Flow out "/1 -> Sum/2
  Flow in/1 -> Sum/1
  Integrator/1 -> p_im/1

== system Project2/Engine/Intercooler ==
  Flow in : Inport
  Flow out : Inport  Port=2
  Integrator : Integrator  InitialCondition=p_amb  LowerSaturationLimit=0
  Product : Product  Inputs=***/  SaturateOnIntegerOverflow=on  OutDataTypeStr=Inherit: Same as first input
  R : Constant  Value=R_air
  Sum : Sum  Inputs=|+-  SaturateOnIntegerOverflow=on
  T_ic : Constant  Value=T_ic
  V_ic : Constant  Value=V_ic
  p_ic : Outport
  wires:
  Integrator/1 -> p_ic/1
  Flow in/1 -> Sum/1
  Flow out/1 -> Sum/2
  R/1 -> Product/2
  T_ic/1 -> Product/3
  Sum/1 -> Product/1
  V_ic/1 -> Product/4
  Product/1 -> Integrator/1

== system Project2/Engine/Lambda dynamics ==
  lam_cyl : Inport
  Gain : Gain  Gain=1/tau_mix
  Integrator : Integrator  InitialCondition=1
  Subtract : Sum  Inputs=+-
  Transport Delay : TransportDelay  DelayTime=tau_d  InitialOutput=1
  lam_bc : Outport
  wires:
  Integrator/1 -> lam_bc/1, Subtract/2
  lam_cyl/1 -> Transport Delay/1
  Transport Delay/1 -> Subtract/1
  Subtract/1 -> Gain/1
  Gain/1 -> Integrator/1

== system Project2/Engine/Lambda sensors ==
  lam : Inport
  Interpreted MATLAB Function : MATLABFcn  MATLABFcn=contToDisc
  Sensor dynamics : Subsystem
  lam_d : Outport
  lam_c : Outport  Port=2
  wires:
  lam/1 -> Sensor dynamics/1(lambda)
  Sensor dynamics/1(lambda_s) -> Interpreted MATLAB Function/1, lam_c/1
  Interpreted MATLAB Function/1 -> lam_d/1

== system Project2/Engine/Luftmassflöde till cylinder ==
  N : Inport
  p_im : Inport  Port=2
  Divide : Product  Inputs=*/
  Divide1 : Product  Inputs=***
  Gain : Gain  Gain=(V_d*n_cyl)/(n_r*R_air)
  Subsystem : Subsystem
  T_im : Constant  Value=T_im
  m_dot_ac : Outport
  wires:
  N/1 -> Divide1/3, Subsystem/1(N)
  p_im/1 -> Divide1/2, Subsystem/2(p_im)
  Subsystem/1(n_vol) -> Divide1/1
  Divide1/1 -> Divide/1
  Divide/1 -> Gain/1
  Gain/1 -> m_dot_ac/1
  T_im/1 -> Divide/2

== system Project2/Engine/Throttle dynamics ==
  AlphaRef : Inport
  Gain : Gain  Gain=1/Tau_th
  Integrator : Integrator
  Subtract : Sum  Inputs=+-
  Alpha : Outport
  wires:
  Integrator/1 -> Alpha/1, Subtract/2
  AlphaRef/1 -> Subtract/1
  Subtract/1 -> Gain/1
  Gain/1 -> Integrator/1

== system Project2/Engine/Trottel FlÃ¶de ==
  p_bef : Inport
  pos : Inport  Port=2
  p_im : Inport  Port=3
  Subsystem1 : Subsystem
  Mass_Flow : Outport
  wires:
  Subsystem1/1(m_dot_at) -> Mass_Flow/1
  pos/1 -> Subsystem1/1(alfa_thr)  "alpha"
  p_im/1 -> Subsystem1/2(p_im)  "p_im"
  p_bef/1 -> Subsystem1/3(p_bef_thr)  "p_bef_thr"

== system Project2/Engine/Turbine ==
  "p_t [Pa] " : Inport
  p_em [Pa] : Inport  Port=2
  w_tc [rad/s] : Inport  Port=3
  Subsystem : Subsystem
  Subsystem6 : Subsystem
  T_em [K] : Constant  Value=T_em
  Tq_t [Nm] : Outport
  m_dot_t [kg/s] : Outport  Port=2
  wires:
  p_em [Pa]/1 -> Subsystem6/4(p_em), Subsystem/2(p03)
  "p_t [Pa] "/1 -> Subsystem6/5(p_t), Subsystem/1(p04)
  T_em [K]/1 -> Subsystem6/2(T_em), Subsystem/3(T_em)
  Subsystem/1(mdot_t) -> Subsystem6/1(mdot_t), m_dot_t [kg/s]/1
  Subsystem6/1(Tq_t) -> Tq_t [Nm]/1
  w_tc [rad/s]/1 -> Subsystem6/6(N_tc), Subsystem6/3(w_tc)

== system Project2/Engine/Turbocharger dynamics ==
  Tq_c [Nm] : Inport
  Tq_t [Nm] : Inport  Port=2
  Damping and friction : Gain  Gain=c_tc_fric  SaturateOnIntegerOverflow=on  OutDataTypeStr=Inherit: Same as input  ParamDataTypeStr=Inherit: Same as input
  Integrator with lower saturation : Integrator  InitialCondition=25e3/30*pi  LimitOutput=on  LowerSaturationLimit="5e3 /  30 * pi"
  Product : Product  Inputs=*/  SaturateOnIntegerOverflow=on  OutDataTypeStr=Inherit: Same as first input
  Sum : Sum  Inputs=+--  SaturateOnIntegerOverflow=on
  turbocharger intertia J : Constant  Value=J_tc
  w_tc [rad/s] : Outport
  wires:
  Integrator with lower saturation/1 -> w_tc [rad/s]/1, Damping and friction/1
  Tq_t [Nm]/1 -> Sum/1
  Tq_c [Nm]/1 -> Sum/2
  turbocharger intertia J/1 -> Product/2
  Sum/1 -> Product/1
  Product/1 -> Integrator with lower saturation/1
  Damping and friction/1 -> Sum/3

== system Project2/Engine/Wastegate ==
  p_t [Pa] : Inport
  wg_pos [0..1] : Inport  Port=2
  p_em [Pa] : Inport  Port=3
  R : Constant  Value=R_exh
  Subsystem1 : Subsystem
  T_em [K] : Constant  Value=T_em
  m_dot_wg [kg/s] : Outport
  wires:
  p_em [Pa]/1 -> Subsystem1/3(p_bef_wg)
  p_t [Pa]/1 -> Subsystem1/2(p_t)
  wg_pos [0..1]/1 -> Subsystem1/1(alfa_wg)  "alpha"
  R/1 -> Subsystem1/5(R_exh)  "R"
  T_em [K]/1 -> Subsystem1/4(T_bef_wg)  "T"
  Subsystem1/1(m_dot_wg) -> m_dot_wg [kg/s]/1

== system Project2/Engine/Wastegate dynamics ==
  u_wg [0..1] : Inport
  Transfer Fcn : TransferFcn  Denominator=[tau_wg 1]
  wg_pos : Outport
  wires:
  u_wg [0..1]/1 -> Transfer Fcn/1  "alpha"
  Transfer Fcn/1 -> wg_pos/1

== system Project2/ECU/Boost Cont/Driver gas pedal interpretation ==
  ped_pos [0..1] : Inport
  N_e [rpm] : Inport  Port=2
  1-D Lookup Table : Lookup_n-D  NumberOfTableDimensions=1  BreakpointsForDimension1=TqEvsNe.Ne  Table=TqEvsNe.TqMAX  RndMeth=Simplest  InputSameDT=on
  1-D Lookup Table2 : Lookup_n-D  NumberOfTableDimensions=1  BreakpointsForDimension1=TqEvsNe.Ne  Table=TqEvsNe.TqMIN  RndMeth=Simplest  InputSameDT=on
  "BMEP -> p_im" : Subsystem
  Constant1 : Constant  Value=0.1
  Constant2 : Constant  Value=0.1
  Gain : Gain  Gain=1/(1-0.9)
  Gain1 : Gain  Gain=1/(1-0.1)
  Product : Product  RndMeth=Zero
  Product1 : Product  RndMeth=Zero
  Subtract : Sum  Inputs=-+
  Subtract1 : Sum  Inputs=+-
  Switch : Switch  Threshold=0.1
  "Tq_ref -> BMEP_ref" : Gain  Gain=2*pi*n_r/(V_D)
  p_im_ref : Outport
  wires:
  ped_pos [0..1]/1 -> Subtract/1, Switch/2, Subtract1/1
  N_e [rpm]/1 -> 1-D Lookup Table2/1, 1-D Lookup Table/1
  Constant1/1 -> Subtract/2
  Subtract/1 -> Gain/1
  Gain/1 -> Product/1
  Constant2/1 -> Subtract1/2
  Subtract1/1 -> Gain1/1
  Gain1/1 -> Product1/1
  1-D Lookup Table/1 -> Product1/2
  1-D Lookup Table2/1 -> Product/2
  Product1/1 -> Switch/1
  Product/1 -> Switch/3
  Switch/1 -> "Tq_ref -> BMEP_ref"/1
  "Tq_ref -> BMEP_ref"/1 -> "BMEP -> p_im"/1(BMEP_ref)
  "BMEP -> p_im"/1(p_im_ref) -> p_im_ref/1

== system Project2/ECU/Boost Cont/Throttle Feed Forward ==
  p_imREF [Pa] : Inport
  N_e [rpm] : Inport  Port=2
  p_icACT [Pa] : Inport  Port=3
  "A_eff " : Subsystem
  Aeff ->alpha_thr : Subsystem
  Gain : Gain  Gain=1/60
  Luftmassflöde till cylinder : Subsystem
  Saturation : Saturate  UpperLimit=1  LowerLimit=0
  alpha_thrFF [0..1] : Outport
  wires:
  p_imREF [Pa]/1 -> "A_eff "/2(p_imREF), Luftmassflöde till cylinder/2(p_im)
  Luftmassflöde till cylinder/1(m_dot_ac) -> "A_eff "/1(mdot_ac)
  p_icACT [Pa]/1 -> "A_eff "/3(pbef)
  "A_eff "/1(A_eff) -> Aeff ->alpha_thr/1(A_eff)
  Aeff ->alpha_thr/1(alpha_thr) -> Saturation/1
  N_e [rpm]/1 -> Gain/1
  Gain/1 -> Luftmassflöde till cylinder/1(N)
  Saturation/1 -> alpha_thrFF [0..1]/1

== system Project2/ECU/Boost Cont/Throttle Feedback including anti-windup ==
  p_imREF [Pa] : Inport
  p_imACT [Pa] : Inport  Port=2
  alpha_thrREFsat [0..1] : Inport  Port=3
  alpha_thrREF [0..1] : Inport  Port=4
  Integrator1 : Integrator  UpperSaturationLimit=5  LowerSaturationLimit=-5
  Scope : Scope
      settings: YMin=-110000  YMax=90000  SaveName=ScopeData14
  Scope2 : Scope
      settings: ShowLegends=on  YMin=-6  YMax=4.5  SaveName=ScopeData21
  Subtract : Sum  Inputs=+-
  Subtract1 : Sum
  Subtract2 : Sum  Inputs=+-
  Subtract3 : Sum  Inputs=-+
  Subtract4 : Sum
  u_FB_wg_Kp : Gain  Gain=KpThr
  u_FB_wg_Kp1 : Gain  Gain=KpThr/TiThr
  u_FB_wg_Kp2 : Gain  Gain=1/TiThr
  alpha_thrFB [0..1] : Outport
  wires:
  p_imACT [Pa]/1 -> Subtract3/1
  p_imREF [Pa]/1 -> Subtract3/2
  Subtract3/1 -> Scope/1, u_FB_wg_Kp/1, u_FB_wg_Kp1/1  "controller error"
  u_FB_wg_Kp/1 -> Subtract4/1
  Subtract4/1 -> alpha_thrFB [0..1]/1
  u_FB_wg_Kp1/1 -> Subtract1/1
  alpha_thrREFsat [0..1]/1 -> Subtract/1, Subtract2/1
  alpha_thrREF [0..1]/1 -> Subtract/2, Subtract2/2
  Subtract2/1 -> u_FB_wg_Kp2/1
  u_FB_wg_Kp2/1 -> Subtract1/2
  Subtract1/1 -> Integrator1/1
  Integrator1/1 -> Subtract4/2
  Subtract/1 -> Scope2/1

== system Project2/ECU/Boost Cont/Waste-gate Feedback including anti-windup ==
  p_imREF [Pa] : Inport
  p_icACT [Pa] : Inport  Port=2
  wgREFsat [0..1] : Inport  Port=3
  wgREF [0..1] : Inport  Port=4
  Add : Sum
  Integrator1 : Integrator  InitialCondition=1
  Scope : Scope  NumInputPorts=2
      settings: ShowLegends=on  YMin=-50000~-0.085  YMax=100000~0  SaveName=ScopeData13
  Subtract1 : Sum
  Subtract2 : Sum  Inputs=+-
  Subtract3 : Sum  Inputs=+-
  Subtract4 : Sum
  Tracking : Gain  Gain=1/TiWg
  a0 : Constant  Value=dP_thrREF
  u_FB_wg_Integral : Gain  Gain=KpWg/TiWg
  u_FB_wg_Proportional : Gain  Gain=KpWg
  wgFB [0..1] : Outport
  wires:
  Integrator1/1 -> Subtract4/2
  Subtract1/1 -> Integrator1/1
  Tracking/1 -> Subtract1/2
  Subtract2/1 -> Scope/2, Tracking/1
  wgREF [0..1]/1 -> Subtract2/2
  wgREFsat [0..1]/1 -> Subtract2/1
  u_FB_wg_Integral/1 -> Subtract1/1
  Subtract4/1 -> wgFB [0..1]/1
  u_FB_wg_Proportional/1 -> Subtract4/1
  Subtract3/1 -> Scope/1, u_FB_wg_Proportional/1, u_FB_wg_Integral/1  "controller error"
  p_icACT [Pa]/1 -> Subtract3/1
  Add/1 -> Subtract3/2
  a0/1 -> Add/2
  p_imREF [Pa]/1 -> Add/1

== system Project2/ECU/Fuel Controller/Luftmassflöde till cylinder ==
  N : Inport
  p_im : Inport  Port=2
  Divide : Product  Inputs=*/
  Divide1 : Product  Inputs=***
  Gain : Gain  Gain=(V_d*n_cyl)/(n_r*R_air)
  Subsystem : Subsystem
  T_im : Constant  Value=T_im
  m_dot_ac : Outport
  wires:
  N/1 -> Subsystem/1(N), Divide1/3
  p_im/1 -> Subsystem/2(p_im), Divide1/2
  Subsystem/1(n_vol) -> Divide1/1
  Divide1/1 -> Divide/1
  Divide/1 -> Gain/1
  Gain/1 -> m_dot_ac/1
  T_im/1 -> Divide/2

== system Project2/ECU/Fuel Controller/PI-reg ==
  Lambda_d : Inport
  Constant : Constant
  Gain : Gain  Gain=KiFuel
  Gain2 : Gain  Gain=KpFuel
  Integrator : Integrator  InitialCondition=1
  Scope1 : Scope
      settings: SaveName=ScopeData11
  Scope2 : Scope
      settings: SaveName=ScopeData15
  Sum : Sum  Inputs=|+++
  Ff : Outport
  wires:
  Integrator/1 -> Gain/1
  Gain/1 -> Sum/2
  Gain2/1 -> Sum/1
  Lambda_d/1 -> Scope1/1, Gain2/1, Integrator/1
  Sum/1 -> Scope2/1, Ff/1
  Constant/1 -> Sum/3

== system Project2/ECU/Fuel Controller/Subsystem ==
  Varvtal : Inport
  m_dotref : Inport  Port=2
  Constant : Constant  Value=t_0
  Divide : Product  Inputs=*/
  Gain3 : Gain  Gain=1/c
  Sum1 : Sum  Inputs=|++
  t_injref : Outport
  wires:
  Sum1/1 -> t_injref/1
  Varvtal/1 -> Divide/2
  Constant/1 -> Sum1/2
  Divide/1 -> Sum1/1
  m_dotref/1 -> Gain3/1
  Gain3/1 -> Divide/1

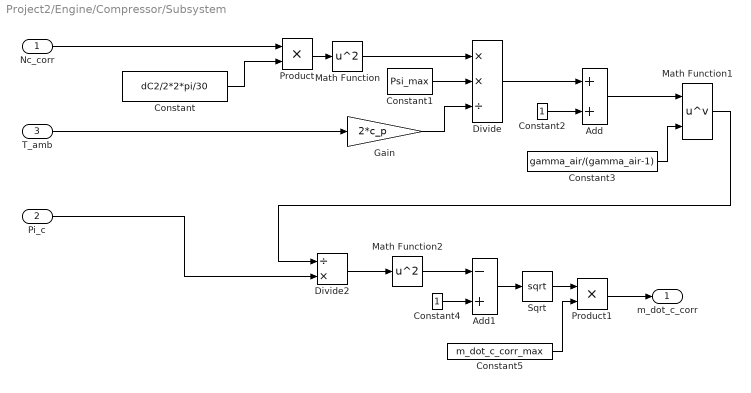
== system Project2/Engine/Compressor/Subsystem ==
  Nc_corr : Inport
  Pi_c : Inport  Port=2
  T_amb : Inport  Port=3
  Add : Sum
  Add1 : Sum  Inputs=-+
  Constant : Constant  Value=dC2/2*2*pi/30
  Constant1 : Constant  Value=Psi_max
  Constant2 : Constant
  Constant3 : Constant  Value=gamma_air/(gamma_air-1)
  Constant4 : Constant
  Constant5 : Constant  Value=m_dot_c_corr_max
  Divide : Product  Inputs=**/
  Divide2 : Product  Inputs=/*
  Gain : Gain  Gain=2*c_p
  Math Function : Math  Operator=square  SaturateOnIntegerOverflow=on
  Math Function1 : Math  Operator=pow  SaturateOnIntegerOverflow=on
  Math Function2 : Math  Operator=square  SaturateOnIntegerOverflow=on
  Product : Product
  Product1 : Product
  Sqrt : Sqrt  SaturateOnIntegerOverflow=on
  m_dot_c_corr : Outport
  wires:
  Constant/1 -> Product/2
  Divide/1 -> Add/1
  Product1/1 -> m_dot_c_corr/1
  Product/1 -> Math Function/1
  Math Function/1 -> Divide/1
  Constant4/1 -> Add1/2
  Gain/1 -> Divide/3
  Pi_c/1 -> Divide2/2
  Math Function1/1 -> Divide2/1
  Constant1/1 -> Divide/2
  Add/1 -> Math Function1/1
  Constant5/1 -> Product1/2
  Divide2/1 -> Math Function2/1
  Add1/1 -> Sqrt/1
  Constant3/1 -> Math Function1/2
  Math Function2/1 -> Add1/1
  Nc_corr/1 -> Product/1
  Constant2/1 -> Add/2
  Sqrt/1 -> Product1/1
  T_amb/1 -> Gain/1

== system Project2/Engine/Compressor/Subsystem2 ==
  m_dot_corr : Inport
  T_amb : Inport  Port=2
  p_amb : Inport  Port=3
  Constant : Constant  Value=p_ref
  Constant1 : Constant  Value=T_ref
  Divide : Product  Inputs=*/
  Divide1 : Product  Inputs=*/
  Product : Product  Inputs=3
  Reciprocal Sqrt : Sqrt  Operator=rSqrt  SaturateOnIntegerOverflow=on
  m_dot_c : Outport
  wires:
  T_amb/1 -> Divide1/1
  p_amb/1 -> Divide/1
  Reciprocal Sqrt/1 -> Product/3
  m_dot_corr/1 -> Product/1
  Constant/1 -> Divide/2
  Divide/1 -> Product/2
  Product/1 -> m_dot_c/1
  Divide1/1 -> Reciprocal Sqrt/1
  Constant1/1 -> Divide1/2

== system Project2/Engine/Compressor/Subsystem3 ==
  eta_c : Inport
  T01 : Inport  Port=2
  Pi_c : Inport  Port=3
  Add : Sum  Inputs=++-
  Constant : Constant  Value=(gamma_air-1)/gamma_air
  Constant1 : Constant
  Divide : Product  Inputs=*/
  Math Function : Math  Operator=pow  SaturateOnIntegerOverflow=on
  Product : Product  RndMeth=Zero
  T_c : Outport
  wires:
  T01/1 -> Divide/1
  eta_c/1 -> Add/2, Divide/2
  Divide/1 -> Product/2
  Pi_c/1 -> Math Function/1
  Constant/1 -> Math Function/2
  Product/1 -> T_c/1
  Add/1 -> Product/1
  Constant1/1 -> Add/3
  Math Function/1 -> Add/1

== system Project2/Engine/Compressor/Subsystem4 ==
  T01 : Inport
  T02 : Inport  Port=2
  mdot_c : Inport  Port=3
  w_tc : Inport  Port=4
  Constant : Constant  Value=0
  Gain : Gain  Gain=cp_air
  MinMax : MinMax  Function=max  Inputs=2
  Product : Product  Inputs=**/  RndMeth=Zero
  Subtract : Sum  Inputs=+-
  Tq_c : Outport
  wires:
  Product/1 -> Gain/1
  Gain/1 -> Tq_c/1
  T02/1 -> Subtract/1
  T01/1 -> Subtract/2
  mdot_c/1 -> Product/2
  w_tc/1 -> Product/3
  MinMax/1 -> Product/1
  Subtract/1 -> MinMax/2
  Constant/1 -> MinMax/1
